simulink model "es728_2simulink"  (R2024b)
settings: Solver=VariableStepAuto  StartTime=0.0  StopTime=10  RelTol=1e-3
values from neighbouring files (symbols this model uses):
  A = [0,   0,   1,    0 ... (first row only)    [es728_1.m]    (also in es728_2.m; es728_3.m)
  a = [1 40 0]    [es728_2.m]
  B = [ 0; 0; 1/mc;  1/(L*mc)]    [es728_1.m]    (also in es728_2.m; es728_3.m)
  b = [1793.9 1793.9*12 1793.9*100]    [es728_2.m]
settings Model: Creator=njsne  LastModifiedBy=njsne

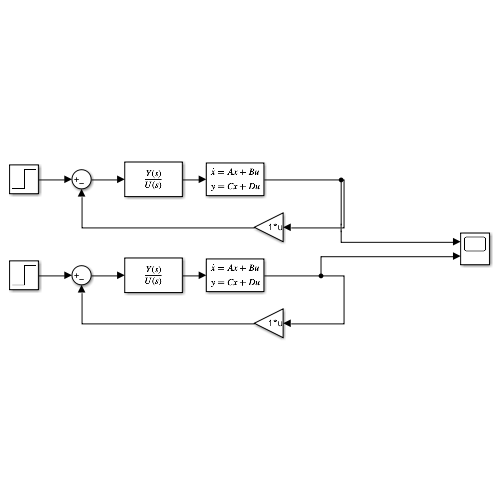
[thumbnail: Simulink's stored preview of the top-level diagram]
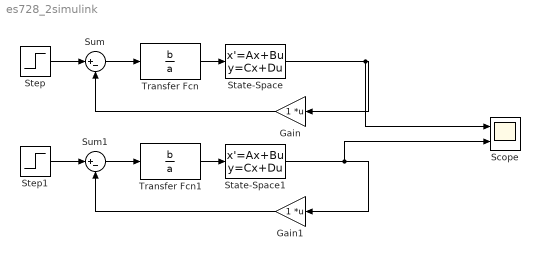
== system es728_2simulink ==
  Gain : Gain  Multiplication=Matrix(K*u)
  Gain1 : Gain  Multiplication=Matrix(K*u)
  Scope : Scope  NumInputPorts=2
  State-Space : StateSpace  A=A  B=B  C=[1 0 0 0]  D=0  InitialCondition=[0.1;0.174533;0;0]
  State-Space1 : StateSpace  A=A  B=B  C=[0 1 0 0]  D=0  InitialCondition=[0.1;0.174533;0;0]
  Step : Step  Time=0  After=0.0  SampleTime=0
  Step1 : Step  Time=0  After=0.0  SampleTime=0
  Sum : Sum  Inputs=|+-
  Sum1 : Sum  Inputs=|+-
  Transfer Fcn : TransferFcn  Numerator=b  Denominator=a
  Transfer Fcn1 : TransferFcn  Numerator=b  Denominator=a
  wires:
  Gain/1 -> Sum/2
  Sum/1 -> Transfer Fcn/1
  Transfer Fcn/1 -> State-Space/1
  Step/1 -> Sum/1
  State-Space/1 -> Gain/1, Scope/1
  Sum1/1 -> Transfer Fcn1/1
  Step1/1 -> Sum1/1
  State-Space1/1 -> Gain1/1, Scope/2
  Gain1/1 -> Sum1/2
  Transfer Fcn1/1 -> State-Space1/1
